simulink model "Testbench_slx_Updated_Presentation"  (R2021a)
settings: Solver=FixedStepAuto  StartTime=0.0  StopTime=0.3  FixedStep=1e-5  RelTol=1e-3
undefined symbols (not defined in the file): D1, Delta
libraries: spsIGBTDiodeLib x52, spsDiodeLib x28, spsSeriesRLCBranchLib x27, spsVariableInductorLib x18, spsGroundLib x7, spsThreePhaseTransformerTwoWindingsLib x6, spsThreePhaseVIMeasurementLib x6, spsAlphaBetaZerotodq0Lib x4, spsVariableCapacitorLib x3, spsVariableResistorLib x3, spsDCVoltageSourceLib x2, pid_lib x2
settings Model: Creator=sjpra  LastModifiedBy=tanmoyera
settings SolverCC: AlgebraicLoopSolver=TrustRegion
settings DebuggingCC: SFMachineParentedDataDiag=warning

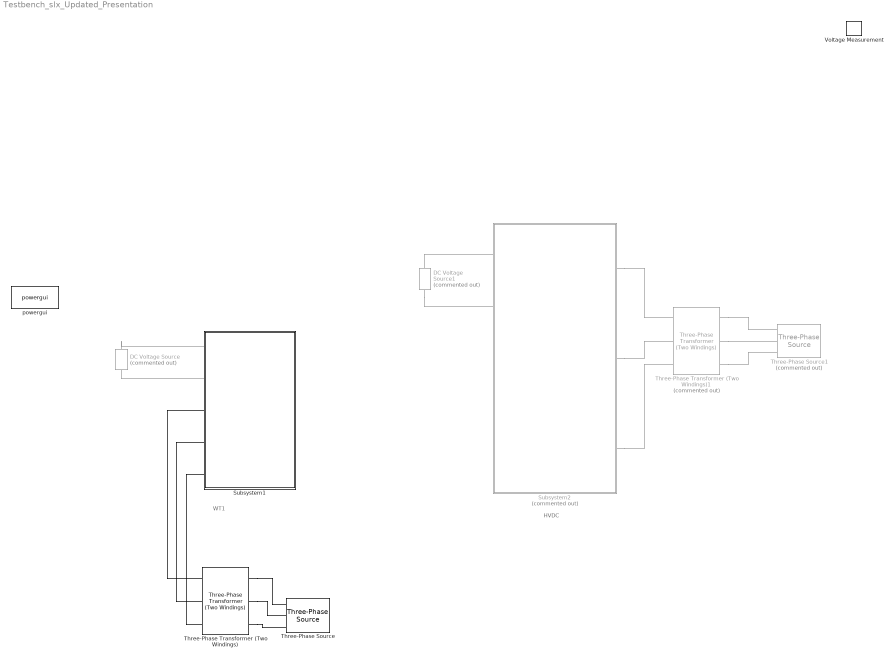
== system Testbench_slx_Updated_Presentation ==
  note: HVDC
  note: WT1
  DC Voltage Source : spsDCVoltageSourceLib/DC Voltage Source  Commented=on  Amplitude=40  Measurements=None
  DC Voltage Source1 : spsDCVoltageSourceLib/DC Voltage Source  Commented=on  Amplitude=40  Measurements=None
  Subsystem1 : Subsystem
  Subsystem2 : Subsystem  Commented=on
  Three-Phase Transformer (Two Windings) : spsThreePhaseTransformerTwoWindingsLib/Three-Phase Transformer (Two Windings)  Winding1Connection=Yg  Winding2Connection=Yg  CoreType=Three single-phase transformers  SetSaturation=off  Hysteresis=off  DataFile='hysteresis'  SetInitialFlux=off  Measurements=None  UNITS=pu  NominalPower=[ 1e3 , 50 ]  Winding1=[ 25 , 0.002 , 0.08 ]  Winding2=[ 400 , 0.002 , 0.08 ]  Rm=500  Lm=500  L0=0.5  Saturation=[ 0,0 ; 0.0024,1.2 ; 1.0,1.52 ]  InitialFluxes=[ 0.8 , -0.8 , 0.7 ]  BreakLoop=off  DiscreteSolver=Trapezoidal iterative  DataType=off  TransfoNumber=1
  Three-Phase Transformer (Two Windings)1 : spsThreePhaseTransformerTwoWindingsLib/Three-Phase Transformer (Two Windings)  Commented=on  Winding1Connection=Yg  Winding2Connection=Yg  CoreType=Three single-phase transformers  SetSaturation=off  Hysteresis=off  DataFile='hysteresis'  SetInitialFlux=off  Measurements=None  UNITS=pu  NominalPower=[ 250e6 , 50 ]  Winding1=[ 25 , 0.002 , 0.08 ]  Winding2=[ 400 , 0.002 , 0.08 ]  Rm=500  Lm=500  L0=0.5  Saturation=[ 0,0 ; 0.0024,1.2 ; 1.0,1.52 ]  InitialFluxes=[ 0.8 , -0.8 , 0.7 ]  BreakLoop=off  DiscreteSolver=Trapezoidal iterative  DataType=off  TransfoNumber=1
  Three-Phase Source : spsThreePhaseSourceLib/Three-Phase Source  InternalConnection=Yg  VoltagePhases=off  Voltage=25e3  PhaseAngle=0  Voltage_phases=[25e3 25e3 25e3]/sqrt(3)  PhaseAngles_phases=[0 -120 +120]  Frequency=50  NonIdealSource=on  SpecifyImpedance=off  Resistance=0.8929  Inductance=16.58e-3  ShortCircuitLevel=100e6  BaseVoltage=25e3  XRratio=7  BusType=swing  Pref=10e3  Qref=0  Prefabc=[10e3, 10e3, 10e3]  Qrefabc=[0, 0, 0]  Qmin=-inf  Qmax=inf
  Three-Phase Source1 : spsThreePhaseSourceLib/Three-Phase Source  Commented=on  InternalConnection=Yg  VoltagePhases=off  Voltage=25e3  PhaseAngle=0  Voltage_phases=[25e3 25e3 25e3]/sqrt(3)  PhaseAngles_phases=[0 -120 +120]  Frequency=50  NonIdealSource=on  SpecifyImpedance=off  Resistance=0.8929  Inductance=16.58e-3  ShortCircuitLevel=100e6  BaseVoltage=25e3  XRratio=7  BusType=swing  Pref=10e3  Qref=0  Prefabc=[10e3, 10e3, 10e3]  Qrefabc=[0, 0, 0]  Qmin=-inf  Qmax=inf
  Voltage Measurement : spsVoltageMeasurementLib/Voltage Measurement  PhasorSimulation=off  OutputType=Complex  PSBequivalent=0
  powergui : spspowerguiLib/powergui  Priority=1  SimulationMode=Discrete  SampleTime=1e-6  frequency=60  Iterations=50  frequencyindice=0  Pbase=1e3  ErrMax=1e-4  UnitsV=V  UnitsW=W  buscounter=0  FunctionMessages=off  echomessages=off  EnableUseOfTLC=off  CurrentSourceSwitches=off  DisableSnubberDevices=off  DisableRonSwitches=off  DisableVfSwitches=off  DisplayEquations=off  AutomaticDiscreteSolvers=off  SolverType=Tustin/Backward Euler (TBE)  Interpol=off  ExternalGateDelay=off  methode=off  Ts=100  x0status=blocks  SPID=on  SwTol=0  HookPort=off  NonlinearTolerance=1e-4  nMaxIteration=100  ContinueOnMaxIteration=off  RestoreLinks=warning  ResistiveCurrentMeasurement=off  Frange=[0:2:500]  Ylog=off  Xlog=on  ShowGrid=off  save=off  variable=ZData  structure=0  ZoomFFT=off  StartTime=0.0  cycles=1  DisplayStyle=1  fundamental=60  FreqAxis=off  MaxFrequency=1000  frequencyindicesteady=1  RmsSteady=1  display=off
  connections:
  DC Voltage Source/RConn1 -- Subsystem1/LConn1
  DC Voltage Source/LConn1 -- Subsystem1/LConn2
  DC Voltage Source1/RConn1 -- Subsystem2/LConn1
  DC Voltage Source1/LConn1 -- Subsystem2/LConn2
  Subsystem1/LConn3 -- Three-Phase Transformer (Two Windings)/LConn1
  Subsystem1/LConn4 -- Three-Phase Transformer (Two Windings)/LConn2
  Subsystem1/LConn5 -- Three-Phase Transformer (Two Windings)/LConn3
  Three-Phase Transformer (Two Windings)/RConn1 -- Three-Phase Source/RConn1
  Three-Phase Transformer (Two Windings)/RConn2 -- Three-Phase Source/RConn2
  Three-Phase Transformer (Two Windings)/RConn3 -- Three-Phase Source/RConn3
  Subsystem2/RConn1 -- Three-Phase Transformer (Two Windings)1/LConn1
  Subsystem2/RConn2 -- Three-Phase Transformer (Two Windings)1/LConn2
  Subsystem2/RConn3 -- Three-Phase Transformer (Two Windings)1/LConn3
  Three-Phase Transformer (Two Windings)1/RConn1 -- Three-Phase Source1/RConn1
  Three-Phase Transformer (Two Windings)1/RConn2 -- Three-Phase Source1/RConn2
  Three-Phase Transformer (Two Windings)1/RConn3 -- Three-Phase Source1/RConn3

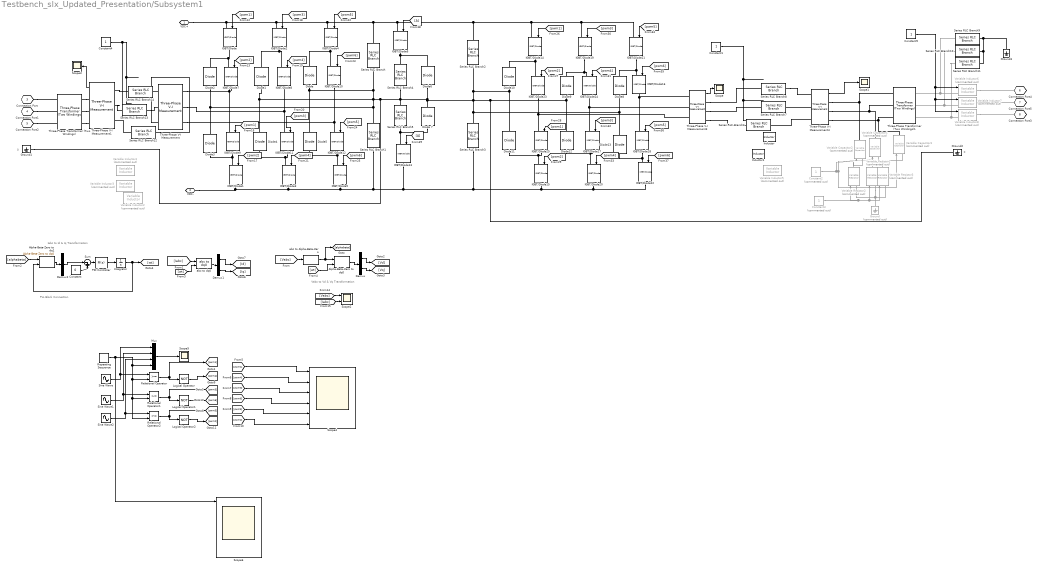
== system Testbench_slx_Updated_Presentation/Subsystem1 ==
  note: 0
  note: 0
  note: Iabc to Id & Iq Transformation
  note: Vabc to Vd & Vq Transformation
  note: PLL Block Connection
  Alpha-Beta-Zero to dq0 : spsAlphaBetaZerotodq0Lib/Alpha-Beta-Zero to dq0  Alignment=90 degrees behind phase A axis
      settings: SourceProductBaseCode=PS
  Alpha-Beta-Zero to dq1 : spsAlphaBetaZerotodq0Lib/Alpha-Beta-Zero to dq0  Alignment=90 degrees behind phase A axis
      settings: SourceProductBaseCode=PS
  Constant : Constant  Value=0
  Constant1 : Constant
  Constant2 : Constant  Commented=on
  Constant3 : Constant  Commented=on
  Constant4 : Constant
  Constant5 : Constant
  Demux : Demux  Outputs=2
  Demux1 : Demux  Outputs=2
  Demux2 : Demux  Outputs=1
  Diode{,1..6,8..13} (13 alike) : spsDiodeLib/Diode  Ron=0.001  Lon=0  Vf=0.8  IC=0  UseSnubber=0  Rs=500  Cs=250e-9  Measurements=off
  Diode 7 : spsDiodeLib/Diode  Ron=0.001  Lon=0  Vf=0.8  IC=0  UseSnubber=0  Rs=500  Cs=250e-9  Measurements=off
  Ground : spsGroundLib/Ground  Commented=on  LConnTagsString=a
  Ground1 : spsGroundLib/Ground  LConnTagsString=a
  Ground2 : spsGroundLib/Ground  LConnTagsString=a
  Ground3 : spsGroundLib/Ground  LConnTagsString=a
  IGBT/Diode{,1..25} (26 alike) : spsIGBTDiodeLib/IGBT//Diode  Ron=1e-3  Rs=1e5  Cs=inf  Measurements=off
  Inductor : fl_lib/Electrical/Electrical Elements/Inductor  l=1e-6 H  r=0 Ohm  g=1e-9 1/Ohm  i_specify=off  i_priority=None  i=0 A  i_nominal_specify=off  i_nominal_unit=A  i_nominal_value=1  v_specify=off  v_priority=None  v=0 V  v_nominal_specify=off  v_nominal_unit=V  v_nominal_value=1  i_L_specify=off  i_L_priority=High  i_L=0 A  i_L_nominal_specify=off  i_L_nominal_unit=A  i_L_nominal_value=1
  Inductor1 : ee_lib/Passive/Inductor  l=1e-6 H  L_tol=20  enable_L_tol=0  tol_distribution=1  nSigma=4  r=0 Ohm  g=1e-9 1/Ohm  enable_operating_limits=0  operating_limit_action=2  max_working_current=1 A  power_rating=1 W  enable_faults=0  fault_action=1  lambdaPercent=50  k_faulted=0.9999  turnsShort=0  openCct=0  groundShort=0  groundShortG=0 1/Ohm  tau_fault=1e-3 s  enable_temporal_fault=0  t_fault=1 s  enable_behavioral_fault=0  max_permissible_voltage=100 V  n_fail_on_voltage=1  max_permissible_current=1 A  t_fail_on_current=1 s  i_L_specify=off  i_L_priority=High  i_L=0 A  i_L_nominal_specify=off  i_L_nominal_unit=A  i_L_nominal_value=1
  Integrator : Integrator
  Logical Operator : Logic  Operator=NOT  AllPortsSameDT=off  OutDataTypeStr=boolean
  Logical Operator1 : Logic  Operator=NOT  AllPortsSameDT=off  OutDataTypeStr=boolean
  Logical Operator2 : Logic  Operator=NOT  AllPortsSameDT=off  OutDataTypeStr=boolean
  Mux : Mux
  PID Controller : pid_lib/PID Controller  Controller=PI  Form=Parallel  TimeDomain=Continuous-time  UseExternalTs=off  SampleTime=-1  IntegratorMethod=Forward Euler  FilterMethod=Forward Euler  ControllerParametersSource=internal  P=10  I=50000  D=0  UseFilter=on  N=100  TunerSelectOption=Transfer Function Based (PID Tuner App)  InitialConditionSource=internal  InitialConditionForIntegrator=0  InitialConditionForFilter=0  DifferentiatorICPrevScaledInput=0  ExternalReset=none  TrackingMode=off  Kt=1  LimitOutput=off  SatLimitsSource=internal  UpperSaturationLimit=inf  LowerSaturationLimit=-inf  LinearizeAsGain=on  AntiWindupMode=none  Kb=1  POutMin=[]  POutMax=[]  IOutMin=[]  IOutMax=[]  DOutMin=[]  DOutMax=[]  NOutMin=[]  NOutMax=[]  SumOutMin=[]  SumOutMax=[]  SaturationOutMin=[]  SaturationOutMax=[]  PParamMin=[]  PParamMax=[]  IParamMin=[]  IParamMax=[]  DParamMin=[]  DParamMax=[]  NParamMin=[]  NParamMax=[]  KbParamMin=[]  KbParamMax=[]  KtParamMin=[]  KtParamMax=[]  KbOutMin=[]  KbOutMax=[]  KtOutMin=[]  KtOutMax=[]  IntegratorOutMin=[]  IntegratorOutMax=[]  FilterOutMin=[]  FilterOutMax=[]  SumI1OutMin=[]  SumI1OutMax=[]  SumI2OutMin=[]  SumI2OutMax=[]  SumI3OutMin=[]  SumI3OutMax=[]  SumI4OutMin=[]  SumI4OutMax=[]  SumDOutMin=[]  SumDOutMax=[]  DifferentiatorOutMin=[]  DifferentiatorOutMax=[]  FilterDiffOutCoefMin=[]  FilterDiffOutCoefMax=[]  ReciprocalOutMin=[]  ReciprocalOutMax=[]  SumDenOutMin=[]  SumDenOutMax=[]  SumNumOutMin=[]  SumNumOutMax=[]  DivideOutMin=[]  DivideOutMax=[]  UdiffTsProdOutMin=[]  UdiffTsProdOutMax=[]  NTsProdOutMin=[]  NTsProdOutMax=[]  UintegralTsProdOutMin=[]  UintegralTsProdOutMax=[]  UngainTsProdOutMin=[]  UngainTsProdOutMax=[]  IntegratorContinuousStateAttributes=''  IntegratorStateMustResolveToSignalObject=off  IntegratorRTWStateStorageClass=Auto  FilterContinuousStateAttributes=''  FilterStateMustResolveToSignalObject=off  FilterRTWStateStorageClass=Auto  ParallelPVariant=InternalParameters  IdealPVariant=Disabled  IVariant=InternalParameters  DVariant=Disabled  IntegratorVariant=Continuous  SatVariant=Disabled  AWVariant=Passthrough  PCopyVariant=Disabled  TRVariant=Disabled  FdbkBlocksVariant=Forward  IdealPFdbkVariant=Disabled  SatFdbkVariant=Disabled  DerivativeFilterVariant=Disabled  NVariant=Disabled  NCopyVariant=Disabled_SignalSpec  FilterICVariant=Disabled  IntegratorICVariant=InternalICs  ExternalResetVariant=Disabled  TRSumVariant=Passthrough  SumFdbkVariant=Disabled  SumVariant=Sum_PI  TsampFilterVariant=InternalTs  TsampNgainVariant=Passthrough  TsampIntegralVariant=Passthrough  ExternalSaturationOutDataTypeStr=Inherit: Same as second input
  Relational Operator : RelationalOperator  OutDataTypeStr=boolean  RndMeth=Simplest
  Relational Operator1 : RelationalOperator  OutDataTypeStr=boolean  RndMeth=Simplest
  Relational Operator2 : RelationalOperator  OutDataTypeStr=boolean  RndMeth=Simplest
  Repeating Sequence : simulink/Sources/Repeating Sequence  rep_seq_t=[0 1 2 3]*[1/6000]  rep_seq_y=[0 1 -1 0]
  Scope{,1,3,5} (4 alike) : Scope
  Scope2 : Scope  NumInputPorts=2
  Scope4 : Scope  NumInputPorts=6
  Scope6 : Scope  NumInputPorts=6
  Series RLC Branch{,1..3} (4 alike) : spsSeriesRLCBranchLib/Series RLC Branch  LConnTagsString=__new0  RConnTagsString=__new0  BranchType=C  Resistance=1  Inductance=1e-3  SetiL0=off  InitialCurrent=0  Capacitance=26e-6  Setx0=off  InitialVoltage=0  Measurements=None
  Series RLC Branch10 : spsSeriesRLCBranchLib/Series RLC Branch  LConnTagsString=__new0  RConnTagsString=__new0  BranchType=R  Resistance=1e6  Inductance=1e-3  SetiL0=off  InitialCurrent=0  Capacitance=1e-6  Setx0=off  InitialVoltage=0  Measurements=None
  Series RLC Branch11 : spsSeriesRLCBranchLib/Series RLC Branch  LConnTagsString=__new0  RConnTagsString=__new0  BranchType=R  Resistance=1e6  Inductance=1e-3  SetiL0=off  InitialCurrent=0  Capacitance=1e-6  Setx0=off  InitialVoltage=0  Measurements=None
  Series RLC Branch{6..8,12..14} (6 alike) : spsSeriesRLCBranchLib/Series RLC Branch  LConnTagsString=__new0  RConnTagsString=__new0  BranchType=L  Resistance=1  Inductance=1e-3  SetiL0=off  InitialCurrent=0  Capacitance=1e-6  Setx0=off  InitialVoltage=0  Measurements=None
  Series RLC Branch4 : spsSeriesRLCBranchLib/Series RLC Branch  LConnTagsString=__new0  RConnTagsString=__new0  BranchType=R  Resistance=1  Inductance=1e-3  SetiL0=off  InitialCurrent=0  Capacitance=1e-6  Setx0=off  InitialVoltage=0  Measurements=None
  Series RLC Branch5 : spsSeriesRLCBranchLib/Series RLC Branch  LConnTagsString=__new0  RConnTagsString=__new0  BranchType=R  Resistance=1  Inductance=1e-3  SetiL0=off  InitialCurrent=0  Capacitance=1e-6  Setx0=off  InitialVoltage=0  Measurements=None
  Series RLC Branch9 : spsSeriesRLCBranchLib/Series RLC Branch  LConnTagsString=__new0  RConnTagsString=__new0  BranchType=R  Resistance=1e6  Inductance=1e-3  SetiL0=off  InitialCurrent=0  Capacitance=1e-6  Setx0=off  InitialVoltage=0  Measurements=None
  Sine Wave : Sin  Frequency=2*pi*50  SampleTime=0
  Sine Wave1 : Sin  Frequency=2*pi*50  Phase=2*pi/3  SampleTime=0
  Sine Wave2 : Sin  Frequency=2*pi*50  Phase=-2*pi/3  SampleTime=0
  Sum : Sum  Inputs=|-+
  Three-Phase Transformer (Two Windings) : spsThreePhaseTransformerTwoWindingsLib/Three-Phase Transformer (Two Windings)  Winding1Connection=Delta (D1)  Winding2Connection=Yg  CoreType=Three single-phase transformers  SetSaturation=off  Hysteresis=off  DataFile='hysteresis'  SetInitialFlux=off  Measurements=None  UNITS=pu  NominalPower=[ 1e3 , 50 ]  Winding1=[ 735e3 , 0.002 , 0.08 ]  Winding2=[ 315e3 , 0.002 , 0.08 ]  Rm=500  Lm=500  L0=0.5  Saturation=[ 0,0 ; 0.0024,1.2 ; 1.0,1.52 ]  InitialFluxes=[ 0.8 , -0.8 , 0.7 ]  BreakLoop=off  DiscreteSolver=Trapezoidal iterative  DataType=off  TransfoNumber=1
  Three-Phase Transformer (Two Windings)1 : spsThreePhaseTransformerTwoWindingsLib/Three-Phase Transformer (Two Windings)  Winding1Connection=Yg  Winding2Connection=Delta (D1)  CoreType=Three single-phase transformers  SetSaturation=off  Hysteresis=off  DataFile='hysteresis'  SetInitialFlux=off  Measurements=None  UNITS=pu  NominalPower=[ 1e3 , 50 ]  Winding1=[ 735e3 , 0.002 , 0.08 ]  Winding2=[ 315e3 , 0.002 , 0.08 ]  Rm=500  Lm=500  L0=0.5  Saturation=[ 0,0 ; 0.0024,1.2 ; 1.0,1.52 ]  InitialFluxes=[ 0.8 , -0.8 , 0.7 ]  BreakLoop=off  DiscreteSolver=Trapezoidal iterative  DataType=off  TransfoNumber=1
  Three-Phase V-I Measurement : spsThreePhaseVIMeasurementLib/Three-Phase V-I Measurement  VoltageMeasurement=no  SetLabelV=off  LabelV=Vabc  Vpu=off  VpuLL=off  CurrentMeasurement=yes  SetLabelI=on  LabelI=IRYB  Ipu=on  Pbase=1e3  Vbase=25  OutputType=Complex  PhasorSimulation=off  PSBequivalent=0
  Three-Phase V-I Measurement1 : spsThreePhaseVIMeasurementLib/Three-Phase V-I Measurement  VoltageMeasurement=phase-to-phase  SetLabelV=off  LabelV=Vabc  Vpu=off  VpuLL=on  CurrentMeasurement=no  SetLabelI=off  LabelI=IRYB  Ipu=off  Pbase=100e6  Vbase=25  OutputType=Complex  PhasorSimulation=off  PSBequivalent=0
  Three-Phase V-I Measurement3 : spsThreePhaseVIMeasurementLib/Three-Phase V-I Measurement  VoltageMeasurement=no  SetLabelV=off  LabelV=Vabc  Vpu=off  VpuLL=off  CurrentMeasurement=yes  SetLabelI=off  LabelI=IRYB  Ipu=off  Pbase=100e6  Vbase=500e3  OutputType=Complex  PhasorSimulation=off  PSBequivalent=0
  Three-Phase V-I Measurement4 : spsThreePhaseVIMeasurementLib/Three-Phase V-I Measurement  VoltageMeasurement=phase-to-phase  SetLabelV=off  LabelV=Vabc  Vpu=off  VpuLL=off  CurrentMeasurement=no  SetLabelI=off  LabelI=IRYB  Ipu=off  Pbase=100e6  Vbase=500e3  OutputType=Complex  PhasorSimulation=off  PSBequivalent=0
  Variable Capacitor1 : spsVariableCapacitorLib/Variable Capacitor  Commented=on  methode=Backward Euler  Cabsmin=235e-6  Initialize=off  vC0=0  C0=1e-6  iC0=0
      settings: SourceProductBaseCode=PS
  Variable Capacitor2 : spsVariableCapacitorLib/Variable Capacitor  Commented=on  methode=Backward Euler  Cabsmin=235e-6  Initialize=off  vC0=0  C0=1e-6  iC0=0
      settings: SourceProductBaseCode=PS
  Variable Capacitor3 : spsVariableCapacitorLib/Variable Capacitor  Commented=on  methode=Backward Euler  Cabsmin=235e-6  Initialize=off  vC0=0  C0=1e-6  iC0=0
      settings: SourceProductBaseCode=PS
  Variable Inductor{2..8} (7 alike) : spsVariableInductorLib/Variable Inductor  Commented=on  methode=Trapezoidal  Labsmin=0.1e-3  Initialize=off  iL0=0  L0=1e-3  Vl0=0
      settings: SourceProductBaseCode=PS
  Variable Resistor1 : spsVariableResistorLib/Variable Resistor  Commented=on  Rabsmin=0.3
      settings: SourceProductBaseCode=PS
  Variable Resistor2 : spsVariableResistorLib/Variable Resistor  Commented=on  Rabsmin=0.3
      settings: SourceProductBaseCode=PS
  Variable Resistor3 : spsVariableResistorLib/Variable Resistor  Commented=on  Rabsmin=0.3
      settings: SourceProductBaseCode=PS
  abc to Alpha-Beta-Zero : spsabctoAlphaBetaZeroLib/abc to Alpha-Beta-Zero
      settings: SourceProductBaseCode=PS
  abc to dq0 : spsabctodq0Lib/abc to dq0  Alignment=90 degrees behind phase A axis
  VDC+ : PMIOPort  Side=Left
  VDC- : PMIOPort  Port=2  Side=Left
  Connection Port : PMIOPort  Tag=PMCPort  Port=3  Side=Left
  Connection Port1 : PMIOPort  Tag=PMCPort  Port=4  Side=Left
  Connection Port2 : PMIOPort  Tag=PMCPort  Port=5  Side=Left
  Connection Port4 : PMIOPort  Tag=PMCPort  Port=6  Side=Right
  Connection Port5 : PMIOPort  Tag=PMCPort  Port=7  Side=Right
  Connection Port3 : PMIOPort  Tag=PMCPort  Port=8  Side=Right
  wires:
  [pwm6] -> IGBT/Diode5/1
  [pwm6] -> IGBT/Diode10/1
  [pwm1] -> IGBT/Diode/1
  [pwm2] -> IGBT/Diode1/1
  [pwm1] -> IGBT/Diode9/1
  [pwm4] -> IGBT/Diode3/1
  [pwm2] -> IGBT/Diode7/1
  [pwm3] -> IGBT/Diode2/1
  [pwm5] -> IGBT/Diode4/1
  [pwm4] -> IGBT/Diode8/1
  [pwm3] -> IGBT/Diode11/1
  [pwm5] -> IGBT/Diode12/1
  [pwm5] -> IGBT/Diode18/1
  [pwm3] -> IGBT/Diode17/1
  [pwm4] -> IGBT/Diode24/1
  [pwm5] -> IGBT/Diode21/1
  [pwm3] -> IGBT/Diode19/1
  [pwm2] -> IGBT/Diode23/1
  [pwm4] -> IGBT/Diode20/1
  [pwm1] -> IGBT/Diode25/1
  [pwm2] -> IGBT/Diode15/1
  [pwm1] -> IGBT/Diode14/1
  [pwm6] -> IGBT/Diode16/1
  [pwm6] -> IGBT/Diode22/1
  Three-Phase V-I Measurement3/1 -> Scope/1
  Three-Phase V-I Measurement4/1 -> Scope1/1
  abc to Alpha-Beta-Zero/1 -> Alpha-Beta-Zero to dq0/1, [alphabeta]
  [Vabc] -> abc to Alpha-Beta-Zero/1
  Alpha-Beta-Zero to dq0/1 -> Demux/1
  Demux/2 -> [Vq]
  [Iabc] -> abc to dq0/1
  abc to dq0/1 -> Demux1/1
  Demux1/2 -> [Iq]
  [alphabeta] -> Alpha-Beta-Zero to dq1/1
  Alpha-Beta-Zero to dq1/1 -> Demux2/1
  Demux2/1 -> Sum/1
  Constant/1 -> Sum/2
  Sum/1 -> PID Controller/1
  PID Controller/1 -> Integrator/1
  Integrator/1 -> [wt], Alpha-Beta-Zero to dq1/2
  [wt] -> abc to dq0/2
  [wt] -> Alpha-Beta-Zero to dq0/2
  [Vabc] -> Scope2/1
  [Iabc] -> Scope2/2
  Three-Phase V-I Measurement1/1 -> Scope3/1
  Demux/1 -> [Vd]
  Demux1/1 -> [Id]
  [A] -> IGBT/Diode6/1
  [A] -> IGBT/Diode13/1
  [pwm6] -> Scope4/4
  [pwm4] -> Scope4/2
  Repeating Sequence/1 -> Scope6/1, Relational Operator/2, Relational Operator1/2, Relational Operator2/2, Mux/4
  Sine Wave2/1 -> Mux/3, Relational Operator2/1
  Relational Operator/1 -> Logical Operator/1, [pwm1]
  Logical Operator2/1 -> [pwm2]
  Mux/1 -> Scope5/1
  Logical Operator1/1 -> [pwm6]
  Sine Wave/1 -> Relational Operator/1, Mux/1
  Relational Operator2/1 -> [pwm5], Logical Operator2/1
  Sine Wave1/1 -> Relational Operator1/1, Mux/2
  [pwm5] -> Scope4/5
  [pwm2] -> Scope4/6
  [pwm3] -> Scope4/3
  [pwm1] -> Scope4/1
  Logical Operator/1 -> [pwm4]
  Relational Operator1/1 -> [pwm3], Logical Operator1/1
  Constant1/1 -> ?
  Constant2/1 -> Variable Capacitor3/1, Variable Capacitor1/1, Variable Capacitor2/1
  Constant3/1 -> Variable Resistor3/1, Variable Resistor1/1, Variable Resistor2/1
  Constant4/1 -> ?
  Constant5/1 -> Variable Inductor8/1, Variable Inductor7/1, Variable Inductor6/1
  connections:
  IGBT/Diode9/RConn1 -- Diode3/LConn1 -- IGBT/Diode1/LConn1
  IGBT/Diode2/RConn1 -- Diode1/RConn1 -- IGBT/Diode8/LConn1
  IGBT/Diode7/RConn1 -- IGBT/Diode9/LConn1 -- Three-Phase V-I Measurement/RConn1
  IGBT/Diode1/RConn1 -- VDC-/RConn1 -- IGBT/Diode3/RConn1 -- Series RLC Branch1/RConn1 -- IGBT/Diode13/RConn1 -- Series RLC Branch3/RConn1 -- IGBT/Diode22/RConn1 -- IGBT/Diode20/RConn1 -- IGBT/Diode15/RConn1 -- IGBT/Diode5/RConn1
  IGBT/Diode10/RConn1 -- IGBT/Diode12/LConn1 -- Three-Phase V-I Measurement/RConn3
  IGBT/Diode11/RConn1 -- Diode4/LConn1 -- IGBT/Diode3/LConn1
  IGBT/Diode12/RConn1 -- Diode5/LConn1 -- IGBT/Diode5/LConn1
  IGBT/Diode7/LConn1 -- IGBT/Diode/RConn1 -- Diode2/RConn1
  IGBT/Diode4/RConn1 -- Diode/RConn1 -- IGBT/Diode10/LConn1
  IGBT/Diode11/LConn1 -- IGBT/Diode8/RConn1 -- Three-Phase V-I Measurement/RConn2
  IGBT/Diode6/RConn1 -- Diode6/RConn1 -- Series RLC Branch4/LConn1
  IGBT/Diode13/LConn1 -- Diode 7/LConn1 -- Series RLC Branch5/RConn1
  Diode11/LConn1 -- IGBT/Diode15/LConn1 -- IGBT/Diode25/RConn1
  Diode9/RConn1 -- IGBT/Diode19/RConn1 -- IGBT/Diode24/LConn1
  IGBT/Diode23/RConn1 -- IGBT/Diode25/LConn1 -- Three-Phase V-I Measurement3/LConn3
  IGBT/Diode18/LConn1 -- IGBT/Diode16/RConn1 -- Three-Phase V-I Measurement3/LConn1
  Diode12/LConn1 -- IGBT/Diode20/LConn1 -- IGBT/Diode17/RConn1
  IGBT/Diode/LConn1 -- VDC+/RConn1 -- Series RLC Branch2/LConn1 -- IGBT/Diode14/LConn1 -- IGBT/Diode21/LConn1 -- IGBT/Diode19/LConn1 -- IGBT/Diode6/LConn1 -- Series RLC Branch/LConn1 -- IGBT/Diode4/LConn1 -- IGBT/Diode2/LConn1
  Diode13/LConn1 -- IGBT/Diode18/RConn1 -- IGBT/Diode22/LConn1
  IGBT/Diode14/RConn1 -- IGBT/Diode23/LConn1 -- Diode10/RConn1
  Diode8/RConn1 -- IGBT/Diode21/RConn1 -- IGBT/Diode16/LConn1
  IGBT/Diode17/LConn1 -- Three-Phase V-I Measurement3/LConn2 -- IGBT/Diode24/RConn1
  Three-Phase V-I Measurement/LConn1 -- Series RLC Branch14/RConn1
  Series RLC Branch13/RConn1 -- Three-Phase V-I Measurement/LConn2
  Series RLC Branch12/RConn1 -- Three-Phase V-I Measurement/LConn3
  Three-Phase V-I Measurement1/LConn1 -- Series RLC Branch14/LConn1
  Three-Phase V-I Measurement1/LConn2 -- Series RLC Branch13/LConn1
  Series RLC Branch12/LConn1 -- Three-Phase V-I Measurement1/LConn3
  Three-Phase Transformer (Two Windings)/RConn1 -- Three-Phase V-I Measurement1/RConn1
  Three-Phase Transformer (Two Windings)/RConn2 -- Three-Phase V-I Measurement1/RConn2
  Three-Phase Transformer (Two Windings)/RConn3 -- Three-Phase V-I Measurement1/RConn3
  Three-Phase V-I Measurement4/LConn2 -- Series RLC Branch7/RConn1
  Three-Phase V-I Measurement4/LConn3 -- Series RLC Branch6/RConn1
  Series RLC Branch8/RConn1 -- Three-Phase V-I Measurement4/LConn1
  Three-Phase V-I Measurement4/RConn1 -- Three-Phase Transformer (Two Windings)1/LConn1 -- Variable Capacitor2/RConn1
  Three-Phase V-I Measurement4/RConn2 -- Three-Phase Transformer (Two Windings)1/LConn2 -- Variable Capacitor1/RConn1
  Three-Phase V-I Measurement4/RConn3 -- Variable Capacitor3/RConn1 -- Three-Phase Transformer (Two Windings)1/LConn3
  Connection Port/RConn1 -- Three-Phase Transformer (Two Windings)/LConn1
  Connection Port1/RConn1 -- Three-Phase Transformer (Two Windings)/LConn2
  Connection Port2/RConn1 -- Three-Phase Transformer (Two Windings)/LConn3
  Variable Resistor1/RConn1 -- Variable Capacitor1/LConn1
  Variable Resistor3/RConn1 -- Variable Capacitor3/LConn1
  Variable Resistor2/RConn1 -- Variable Capacitor2/LConn1
  Variable Resistor2/LConn1 -- Variable Resistor3/LConn1 -- Ground/LConn1 -- Variable Resistor1/LConn1
  Diode13/RConn1 -- Diode8/LConn1 -- Diode12/RConn1 -- Diode9/LConn1 -- Ground2/LConn1 -- Series RLC Branch5/LConn1 -- Series RLC Branch4/RConn1 -- Ground1/LConn1 -- Diode3/RConn1 -- Diode2/LConn1 -- Series RLC Branch1/LConn1 -- Diode5/RConn1 -- Diode/LConn1 -- Series RLC Branch/RConn1 -- Diode1/LConn1 -- Diode4/RConn1 -- Diode6/LConn1 -- Diode 7/RConn1 -- Series RLC Branch2/RConn1 -- Diode11/RConn1 -- Diode10/LConn1 -- Series RLC Branch3/LConn1
  Three-Phase V-I Measurement3/RConn1 -- Series RLC Branch8/LConn1
  Three-Phase V-I Measurement3/RConn2 -- Series RLC Branch7/LConn1
  Three-Phase V-I Measurement3/RConn3 -- Series RLC Branch6/LConn1
  Variable Inductor6/LConn1 -- Series RLC Branch9/LConn1 -- Three-Phase Transformer (Two Windings)1/RConn1
  Variable Inductor7/LConn1 -- Series RLC Branch10/LConn1 -- Three-Phase Transformer (Two Windings)1/RConn2
  Variable Inductor8/LConn1 -- Series RLC Branch11/LConn1 -- Three-Phase Transformer (Two Windings)1/RConn3
  Variable Inductor6/RConn1 -- Connection Port4/RConn1
  Variable Inductor7/RConn1 -- Connection Port5/RConn1
  Variable Inductor8/RConn1 -- Connection Port3/RConn1
  Series RLC Branch9/RConn1 -- Series RLC Branch10/RConn1 -- Series RLC Branch11/RConn1 -- Ground3/LConn1

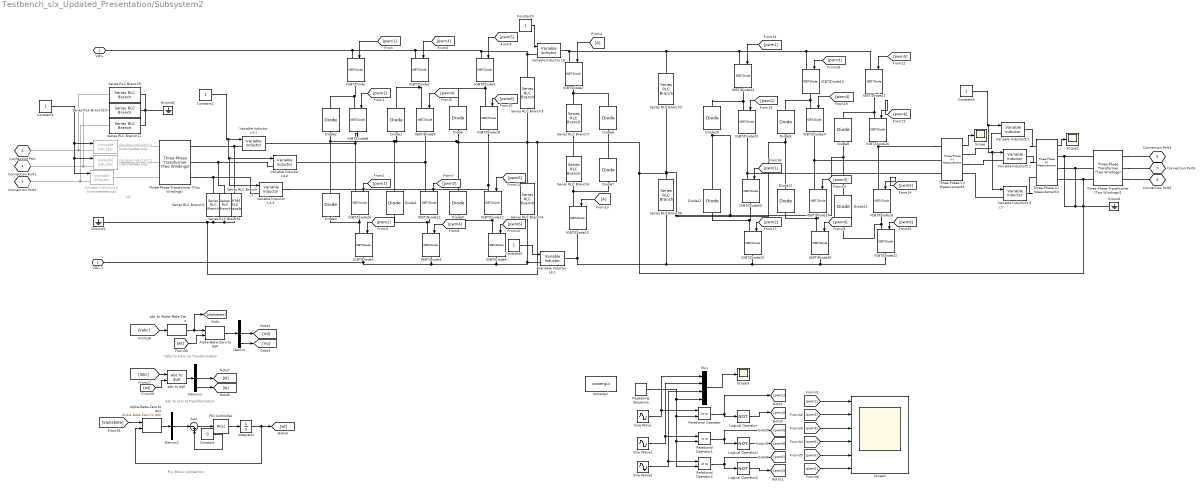
== system Testbench_slx_Updated_Presentation/Subsystem2 ==
  note: L5
  note: L4
  note: L3
  note: Vabc to Vd & Vq Transformation
  note: Iabc to Id & Iq Transformation
  note: PLL Block Connection
  Alpha-Beta-Zero to dq0 : spsAlphaBetaZerotodq0Lib/Alpha-Beta-Zero to dq0  Alignment=90 degrees behind phase A axis
      settings: SourceProductBaseCode=PS
  Alpha-Beta-Zero to dq1 : spsAlphaBetaZerotodq0Lib/Alpha-Beta-Zero to dq0  Alignment=90 degrees behind phase A axis
      settings: SourceProductBaseCode=PS
  Constant : Constant  Value=0
  Constant{1..5} (5 alike) : Constant
  Demux : Demux  Outputs=3
  Demux1 : Demux  Outputs=3
  Demux2 : Demux  Outputs=3
  Diode{,1..13} (14 alike) : spsDiodeLib/Diode  Ron=0.001  Lon=0  Vf=0.8  IC=0  UseSnubber=0  Rs=500  Cs=250e-9  Measurements=off
  Ground : spsGroundLib/Ground  LConnTagsString=a
  Ground1 : spsGroundLib/Ground  LConnTagsString=a
  Ground2 : spsGroundLib/Ground  LConnTagsString=a
  IGBT/Diode{,1..5,7..26} (26 alike) : spsIGBTDiodeLib/IGBT//Diode  Ron=1e-3  Rs=1e5  Cs=inf  Measurements=off
  Integrator : Integrator
  Logical Operator : Logic  Operator=NOT  AllPortsSameDT=off  OutDataTypeStr=boolean
  Logical Operator1 : Logic  Operator=NOT  AllPortsSameDT=off  OutDataTypeStr=boolean
  Logical Operator2 : Logic  Operator=NOT  AllPortsSameDT=off  OutDataTypeStr=boolean
  Mux : Mux
  PID Controller : pid_lib/PID Controller  Controller=PI  Form=Parallel  TimeDomain=Continuous-time  UseExternalTs=off  SampleTime=-1  IntegratorMethod=Forward Euler  FilterMethod=Forward Euler  ControllerParametersSource=internal  P=10  I=50000  D=0  UseFilter=on  N=100  TunerSelectOption=Transfer Function Based (PID Tuner App)  InitialConditionSource=internal  InitialConditionForIntegrator=0  InitialConditionForFilter=0  DifferentiatorICPrevScaledInput=0  ExternalReset=none  TrackingMode=off  Kt=1  LimitOutput=off  SatLimitsSource=internal  UpperSaturationLimit=inf  LowerSaturationLimit=-inf  LinearizeAsGain=on  AntiWindupMode=none  Kb=1  POutMin=[]  POutMax=[]  IOutMin=[]  IOutMax=[]  DOutMin=[]  DOutMax=[]  NOutMin=[]  NOutMax=[]  SumOutMin=[]  SumOutMax=[]  SaturationOutMin=[]  SaturationOutMax=[]  PParamMin=[]  PParamMax=[]  IParamMin=[]  IParamMax=[]  DParamMin=[]  DParamMax=[]  NParamMin=[]  NParamMax=[]  KbParamMin=[]  KbParamMax=[]  KtParamMin=[]  KtParamMax=[]  KbOutMin=[]  KbOutMax=[]  KtOutMin=[]  KtOutMax=[]  IntegratorOutMin=[]  IntegratorOutMax=[]  FilterOutMin=[]  FilterOutMax=[]  SumI1OutMin=[]  SumI1OutMax=[]  SumI2OutMin=[]  SumI2OutMax=[]  SumI3OutMin=[]  SumI3OutMax=[]  SumI4OutMin=[]  SumI4OutMax=[]  SumDOutMin=[]  SumDOutMax=[]  DifferentiatorOutMin=[]  DifferentiatorOutMax=[]  FilterDiffOutCoefMin=[]  FilterDiffOutCoefMax=[]  ReciprocalOutMin=[]  ReciprocalOutMax=[]  SumDenOutMin=[]  SumDenOutMax=[]  SumNumOutMin=[]  SumNumOutMax=[]  DivideOutMin=[]  DivideOutMax=[]  UdiffTsProdOutMin=[]  UdiffTsProdOutMax=[]  NTsProdOutMin=[]  NTsProdOutMax=[]  UintegralTsProdOutMin=[]  UintegralTsProdOutMax=[]  UngainTsProdOutMin=[]  UngainTsProdOutMax=[]  IntegratorContinuousStateAttributes=''  IntegratorStateMustResolveToSignalObject=off  IntegratorRTWStateStorageClass=Auto  FilterContinuousStateAttributes=''  FilterStateMustResolveToSignalObject=off  FilterRTWStateStorageClass=Auto  ParallelPVariant=InternalParameters  IdealPVariant=Disabled  IVariant=InternalParameters  DVariant=Disabled  IntegratorVariant=Continuous  SatVariant=Disabled  AWVariant=Passthrough  PCopyVariant=Disabled  TRVariant=Disabled  FdbkBlocksVariant=Forward  IdealPFdbkVariant=Disabled  SatFdbkVariant=Disabled  DerivativeFilterVariant=Disabled  NVariant=Disabled  NCopyVariant=Disabled_SignalSpec  FilterICVariant=Disabled  IntegratorICVariant=InternalICs  ExternalResetVariant=Disabled  TRSumVariant=Passthrough  SumFdbkVariant=Disabled  SumVariant=Sum_PI  TsampFilterVariant=InternalTs  TsampNgainVariant=Passthrough  TsampIntegralVariant=Passthrough  ExternalSaturationOutDataTypeStr=Inherit: Same as second input
  Relational Operator : RelationalOperator  OutDataTypeStr=boolean  RndMeth=Simplest
  Relational Operator1 : RelationalOperator  OutDataTypeStr=boolean  RndMeth=Simplest
  Relational Operator2 : RelationalOperator  OutDataTypeStr=boolean  RndMeth=Simplest
  Repeating Sequence : simulink/Sources/Repeating Sequence  rep_seq_t=[0 1 2 3]*[1/6000]  rep_seq_y=[0 1 -1 0]
  Scope : Scope
  Scope1 : Scope
  Scope2 : Scope  NumInputPorts=6
  Scope3 : Scope
  Series RLC Branch : spsSeriesRLCBranchLib/Series RLC Branch  LConnTagsString=__new0  RConnTagsString=__new0  BranchType=C  Resistance=1  Inductance=1e-3  SetiL0=off  InitialCurrent=0  Capacitance=1e-6  Setx0=off  InitialVoltage=0  Measurements=None
  Series RLC Branch1 : spsSeriesRLCBranchLib/Series RLC Branch  LConnTagsString=__new0  RConnTagsString=__new0  BranchType=C  Resistance=1  Inductance=1e-3  SetiL0=off  InitialCurrent=0  Capacitance=1e-6  Setx0=off  InitialVoltage=0  Measurements=None
  Series RLC Branch10 : spsSeriesRLCBranchLib/Series RLC Branch  LConnTagsString=__new0  RConnTagsString=__new0  BranchType=R  Resistance=1e6  Inductance=1e-3  SetiL0=off  InitialCurrent=0  Capacitance=1e-6  Setx0=off  InitialVoltage=0  Measurements=None
  Series RLC Branch11 : spsSeriesRLCBranchLib/Series RLC Branch  LConnTagsString=__new0  RConnTagsString=__new0  BranchType=R  Resistance=1e6  Inductance=1e-3  SetiL0=off  InitialCurrent=0  Capacitance=1e-6  Setx0=off  InitialVoltage=0  Measurements=None
  Series RLC Branch2 : spsSeriesRLCBranchLib/Series RLC Branch  LConnTagsString=__new0  RConnTagsString=__new0  BranchType=C  Resistance=1  Inductance=1e-3  SetiL0=off  InitialCurrent=0  Capacitance=1e-6  Setx0=off  InitialVoltage=0  Measurements=None
  Series RLC Branch{3..6} (4 alike) : spsSeriesRLCBranchLib/Series RLC Branch  LConnTagsString=__new0  RConnTagsString=__new0  BranchType=C  Resistance=1  Inductance=1e-3  SetiL0=off  InitialCurrent=0  Capacitance=26e-6  Setx0=off  InitialVoltage=0  Measurements=None
  Series RLC Branch7 : spsSeriesRLCBranchLib/Series RLC Branch  LConnTagsString=__new0  RConnTagsString=__new0  BranchType=R  Resistance=1  Inductance=1e-3  SetiL0=off  InitialCurrent=0  Capacitance=1e-6  Setx0=off  InitialVoltage=0  Measurements=None
  Series RLC Branch8 : spsSeriesRLCBranchLib/Series RLC Branch  LConnTagsString=__new0  RConnTagsString=__new0  BranchType=R  Resistance=1  Inductance=1e-3  SetiL0=off  InitialCurrent=0  Capacitance=1e-6  Setx0=off  InitialVoltage=0  Measurements=None
  Series RLC Branch9 : spsSeriesRLCBranchLib/Series RLC Branch  LConnTagsString=__new0  RConnTagsString=__new0  BranchType=R  Resistance=1e6  Inductance=1e-3  SetiL0=off  InitialCurrent=0  Capacitance=1e-6  Setx0=off  InitialVoltage=0  Measurements=None
  Sine Wave : Sin  Frequency=2*pi*50  SampleTime=0
  Sine Wave1 : Sin  Frequency=2*pi*50  Phase=2*pi/3  SampleTime=0
  Sine Wave2 : Sin  Frequency=2*pi*50  Phase=-2*pi/3  SampleTime=0
  Sum : Sum  Inputs=|-+
  Three-Phase Transformer (Two Windings) : spsThreePhaseTransformerTwoWindingsLib/Three-Phase Transformer (Two Windings)  Winding1Connection=Delta (D1)  Winding2Connection=Y  CoreType=Three single-phase transformers  SetSaturation=off  Hysteresis=off  DataFile='hysteresis'  SetInitialFlux=off  Measurements=None  UNITS=pu  NominalPower=[ 250e6 , 60 ]  Winding1=[ 735e3 , 0.002 , 0.08 ]  Winding2=[ 315e3 , 0.002 , 0.08 ]  Rm=500  Lm=500  L0=0.5  Saturation=[ 0,0 ; 0.0024,1.2 ; 1.0,1.52 ]  InitialFluxes=[ 0.8 , -0.8 , 0.7 ]  BreakLoop=off  DiscreteSolver=Trapezoidal iterative  DataType=off  TransfoNumber=1
  Three-Phase Transformer (Two Windings)1 : spsThreePhaseTransformerTwoWindingsLib/Three-Phase Transformer (Two Windings)  Winding1Connection=Yg  Winding2Connection=Delta (D1)  CoreType=Three single-phase transformers  SetSaturation=off  Hysteresis=off  DataFile='hysteresis'  SetInitialFlux=off  Measurements=None  UNITS=pu  NominalPower=[ 250e6 , 60 ]  Winding1=[ 735e3 , 0.002 , 0.08 ]  Winding2=[ 315e3 , 0.002 , 0.08 ]  Rm=500  Lm=500  L0=0.5  Saturation=[ 0,0 ; 0.0024,1.2 ; 1.0,1.52 ]  InitialFluxes=[ 0.8 , -0.8 , 0.7 ]  BreakLoop=off  DiscreteSolver=Trapezoidal iterative  DataType=off  TransfoNumber=1
  Three-Phase V-I Measurement3 : spsThreePhaseVIMeasurementLib/Three-Phase V-I Measurement  VoltageMeasurement=no  SetLabelV=off  LabelV=Vabc  Vpu=off  VpuLL=off  CurrentMeasurement=yes  SetLabelI=off  LabelI=IRYB  Ipu=off  Pbase=100e6  Vbase=500e3  OutputType=Complex  PhasorSimulation=off  PSBequivalent=0
  Three-Phase V-I Measurement4 : spsThreePhaseVIMeasurementLib/Three-Phase V-I Measurement  VoltageMeasurement=phase-to-phase  SetLabelV=off  LabelV=Vabc  Vpu=off  VpuLL=off  CurrentMeasurement=no  SetLabelI=off  LabelI=IRYB  Ipu=off  Pbase=100e6  Vbase=500e3  OutputType=Complex  PhasorSimulation=off  PSBequivalent=0
  Variable Inductor L4.1 : spsVariableInductorLib/Variable Inductor  methode=Trapezoidal  Labsmin=0.1e-3  Initialize=off  iL0=0  L0=1e-3  Vl0=0
      settings: SourceProductBaseCode=PS
  Variable Inductor L4.2 : spsVariableInductorLib/Variable Inductor  methode=Trapezoidal  Labsmin=0.1e-3  Initialize=off  iL0=0  L0=1e-3  Vl0=0
      settings: SourceProductBaseCode=PS
  Variable Inductor L4.3 : spsVariableInductorLib/Variable Inductor  methode=Trapezoidal  Labsmin=0.1e-3  Initialize=off  iL0=0  L0=1e-3  Vl0=0
      settings: SourceProductBaseCode=PS
  Variable Inductor L6 : spsVariableInductorLib/Variable Inductor  methode=Backward Euler  Labsmin=0.1e-3  Initialize=off  iL0=0  L0=1e-3  Vl0=0
      settings: SourceProductBaseCode=PS
  Variable Inductor L6.1 : spsVariableInductorLib/Variable Inductor  methode=Backward Euler  Labsmin=0.1e-3  Initialize=off  iL0=0  L0=1e-3  Vl0=0
      settings: SourceProductBaseCode=PS
  Variable Inductor5.1 : spsVariableInductorLib/Variable Inductor  methode=Trapezoidal  Labsmin=0.1e-3  Initialize=off  iL0=0  L0=1e-3  Vl0=0
      settings: SourceProductBaseCode=PS
  Variable Inductor5.2 : spsVariableInductorLib/Variable Inductor  methode=Trapezoidal  Labsmin=0.1e-3  Initialize=off  iL0=0  L0=1e-3  Vl0=0
      settings: SourceProductBaseCode=PS
  Variable Inductor5.3 : spsVariableInductorLib/Variable Inductor  methode=Trapezoidal  Labsmin=0.1e-3  Initialize=off  iL0=0  L0=1e-3  Vl0=0
      settings: SourceProductBaseCode=PS
  Variable Inductor5.4 : spsVariableInductorLib/Variable Inductor  Commented=on  methode=Trapezoidal  Labsmin=0.1e-3  Initialize=off  iL0=0  L0=1e-3  Vl0=0
      settings: SourceProductBaseCode=PS
  Variable Inductor5.5 : spsVariableInductorLib/Variable Inductor  Commented=on  methode=Trapezoidal  Labsmin=0.1e-3  Initialize=off  iL0=0  L0=1e-3  Vl0=0
      settings: SourceProductBaseCode=PS
  Variable Inductor5.6 : spsVariableInductorLib/Variable Inductor  Commented=on  methode=Trapezoidal  Labsmin=0.1e-3  Initialize=off  iL0=0  L0=1e-3  Vl0=0
      settings: SourceProductBaseCode=PS
  abc to Alpha-Beta-Zero : spsabctoAlphaBetaZeroLib/abc to Alpha-Beta-Zero
      settings: SourceProductBaseCode=PS
  abc to dq0 : spsabctodq0Lib/abc to dq0  Alignment=90 degrees behind phase A axis
  powergui : spspowerguiLib/powergui  Priority=1  SimulationMode=Continuous  SampleTime=50e-6  frequency=60  Iterations=50  frequencyindice=60  Pbase=100e6  ErrMax=1e-4  UnitsV=kV  UnitsW=MW  buscounter=0  FunctionMessages=off  echomessages=off  EnableUseOfTLC=off  CurrentSourceSwitches=off  DisableSnubberDevices=off  DisableRonSwitches=off  DisableVfSwitches=off  DisplayEquations=off  AutomaticDiscreteSolvers=off  SolverType=Tustin/Backward Euler (TBE)  Interpol=off  ExternalGateDelay=off  methode=off  Ts=100  x0status=blocks  SPID=on  SwTol=0  HookPort=off  NonlinearTolerance=1e-4  nMaxIteration=100  ContinueOnMaxIteration=off  RestoreLinks=warning  ResistiveCurrentMeasurement=off  Frange=[0:2:500]  Ylog=off  Xlog=on  ShowGrid=off  save=off  variable=ZData  structure=0  ZoomFFT=off  StartTime=0.0  cycles=1  DisplayStyle=1  fundamental=60  FreqAxis=off  MaxFrequency=1000  frequencyindicesteady=1  RmsSteady=1  display=off
  VDC- : PMIOPort  Side=Left
  VDC-1 : PMIOPort  Port=2  Side=Left
  Connection Port : PMIOPort  Tag=PMCPort  Port=3  Side=Left
  Connection Port1 : PMIOPort  Tag=PMCPort  Port=4  Side=Left
  Connection Port2 : PMIOPort  Tag=PMCPort  Port=5  Side=Left
  Connection Port3 : PMIOPort  Tag=PMCPort  Port=6  Side=Right
  Connection Port4 : PMIOPort  Tag=PMCPort  Port=7  Side=Right
  Connection Port5 : PMIOPort  Tag=PMCPort  Port=8  Side=Right
  wires:
  Three-Phase V-I Measurement3/1 -> Scope/1
  [pwm1] -> IGBT/Diode/1
  Sum/1 -> PID Controller/1
  Alpha-Beta-Zero to dq0/1 -> Demux/1
  Demux/3 -> [Vq]
  Demux1/3 -> [Iq]
  [Vabc] -> abc to Alpha-Beta-Zero/1
  [alphabeta] -> Alpha-Beta-Zero to dq1/1
  Demux1/2 -> [Id]
  Integrator/1 -> [wt], Alpha-Beta-Zero to dq1/2
  Constant/1 -> Sum/2
  [Iabc] -> abc to dq0/1
  abc to dq0/1 -> Demux1/1
  [wt] -> abc to dq0/2
  [wt] -> Alpha-Beta-Zero to dq0/2
  Demux2/2 -> Sum/1
  PID Controller/1 -> Integrator/1
  abc to Alpha-Beta-Zero/1 -> Alpha-Beta-Zero to dq0/1, [alphabeta]
  Demux/2 -> [Vd]
  Alpha-Beta-Zero to dq1/1 -> Demux2/1
  [pwm2] -> IGBT/Diode8/1
  [pwm1] -> IGBT/Diode26/1
  Three-Phase V-I Measurement4/1 -> Scope1/1
  [pwm2] -> IGBT/Diode1/1
  [pwm3] -> IGBT/Diode2/1
  [pwm4] -> IGBT/Diode9/1
  [pwm4] -> IGBT/Diode3/1
  [pwm5] -> IGBT/Diode4/1
  [pwm3] -> IGBT/Diode11/1
  [pwm5] -> IGBT/Diode12/1
  [pwm6] -> IGBT/Diode5/1
  [A] -> IGBT/Diode7/1
  [A] -> IGBT/Diode13/1
  [pwm1] -> IGBT/Diode14/1
  [pwm2] -> IGBT/Diode23/1
  [pwm1] -> IGBT/Diode25/1
  [pwm2] -> IGBT/Diode15/1
  [pwm3] -> IGBT/Diode19/1
  [pwm4] -> IGBT/Diode24/1
  [pwm4] -> IGBT/Diode20/1
  [pwm3] -> IGBT/Diode17/1
  [pwm5] -> IGBT/Diode21/1
  [pwm6] -> IGBT/Diode16/1
  [pwm5] -> IGBT/Diode18/1
  [pwm6] -> IGBT/Diode22/1
  [pwm6] -> IGBT/Diode10/1
  [pwm6] -> Scope2/4
  [pwm4] -> Scope2/2
  Repeating Sequence/1 -> Relational Operator/2, Relational Operator1/2, Relational Operator2/2, Mux/4
  Sine Wave2/1 -> Mux/3, Relational Operator2/1
  Relational Operator/1 -> Logical Operator/1, [pwm1]
  Logical Operator2/1 -> [pwm2]
  Mux/1 -> Scope3/1
  Logical Operator1/1 -> [pwm6]
  Sine Wave/1 -> Relational Operator/1, Mux/1
  Relational Operator2/1 -> [pwm5], Logical Operator2/1
  Sine Wave1/1 -> Relational Operator1/1, Mux/2
  [pwm5] -> Scope2/5
  [pwm2] -> Scope2/6
  [pwm3] -> Scope2/3
  [pwm1] -> Scope2/1
  Logical Operator/1 -> [pwm4]
  Relational Operator1/1 -> [pwm3], Logical Operator1/1
  Constant2/1 -> Variable Inductor L4.3/1, Variable Inductor L4.2/1, Variable Inductor L4.1/1
  Constant3/1 -> Variable Inductor L6/1
  Constant4/1 -> Variable Inductor L6.1/1
  Constant5/1 -> Variable Inductor5.3/1, Variable Inductor5.2/1, Variable Inductor5.1/1
  Constant1/1 -> Variable Inductor5.6/1, Variable Inductor5.5/1, Variable Inductor5.4/1
  connections:
  IGBT/Diode/LConn1 -- Variable Inductor L6/LConn1 -- Series RLC Branch3/LConn1 -- IGBT/Diode4/LConn1 -- IGBT/Diode2/LConn1 -- VDC-/RConn1
  Series RLC Branch1/LConn1 -- Three-Phase Transformer (Two Windings)/RConn2 -- Variable Inductor L4.2/LConn1
  Series RLC Branch1/RConn1 -- Series RLC Branch/RConn1 -- Series RLC Branch2/RConn1 -- Ground1/LConn1 -- Diode8/LConn1 -- Diode13/RConn1 -- Diode11/RConn1 -- Diode10/LConn1 -- Diode12/RConn1 -- Diode9/LConn1 -- Series RLC Branch5/RConn1 -- Series RLC Branch6/LConn1 -- Three-Phase Transformer (Two Windings)1/LConn2 -- Three-Phase V-I Measurement4/RConn2 -- Three-Phase V-I Measurement4/RConn1 -- Three-Phase Transformer (Two Windings)1/LConn1 -- Three-Phase V-I Measurement4/RConn3 -- Three-Phase Transformer (Two Windings)1/LConn3 -- Ground/LConn1 -- Diode5/RConn1 -- Diode1/LConn1 -- Diode3/RConn1 -- Diode2/LConn1 -- Diode4/RConn1 -- Diode/LConn1 -- Series RLC Branch4/LConn1 -- Series RLC Branch3/RConn1
  Three-Phase Transformer (Two Windings)/RConn3 -- Series RLC Branch2/LConn1 -- Variable Inductor L4.3/LConn1
  IGBT/Diode25/RConn1 -- Diode11/LConn1 -- IGBT/Diode15/LConn1
  IGBT/Diode19/LConn1 -- IGBT/Diode21/LConn1 -- Variable Inductor L6/RConn1 -- IGBT/Diode7/LConn1 -- Series RLC Branch5/LConn1 -- IGBT/Diode14/LConn1
  Three-Phase Transformer (Two Windings)/RConn1 -- Series RLC Branch/LConn1 -- Variable Inductor L4.1/LConn1
  IGBT/Diode1/LConn1 -- IGBT/Diode26/RConn1 -- Diode3/LConn1
  Three-Phase V-I Measurement3/LConn1 -- IGBT/Diode18/LConn1 -- IGBT/Diode16/RConn1
  IGBT/Diode22/LConn1 -- Diode13/LConn1 -- IGBT/Diode18/RConn1
  Variable Inductor L6.1/LConn1 -- Series RLC Branch4/RConn1 -- IGBT/Diode5/RConn1 -- IGBT/Diode3/RConn1 -- IGBT/Diode1/RConn1 -- VDC-1/RConn1
  Series RLC Branch8/RConn1 -- IGBT/Diode13/LConn1 -- Diode7/LConn1
  IGBT/Diode5/LConn1 -- IGBT/Diode12/RConn1 -- Diode5/LConn1
  Variable Inductor5.6/RConn1 -- Three-Phase Transformer (Two Windings)/LConn3
  IGBT/Diode15/RConn1 -- IGBT/Diode22/RConn1 -- IGBT/Diode20/RConn1 -- Series RLC Branch6/RConn1 -- IGBT/Diode13/RConn1 -- Variable Inductor L6.1/RConn1
  Three-Phase V-I Measurement3/LConn2 -- IGBT/Diode17/LConn1 -- IGBT/Diode24/RConn1
  Three-Phase V-I Measurement4/LConn1 -- Variable Inductor5.1/RConn1
  Variable Inductor5.3/RConn1 -- Three-Phase V-I Measurement4/LConn3
  Series RLC Branch7/RConn1 -- Series RLC Branch8/LConn1
  Three-Phase V-I Measurement3/RConn2 -- Variable Inductor5.2/LConn1
  Diode9/RConn1 -- IGBT/Diode19/RConn1 -- IGBT/Diode24/LConn1
  Three-Phase V-I Measurement4/LConn2 -- Variable Inductor5.2/RConn1
  Three-Phase Transformer (Two Windings)1/RConn3 -- Connection Port5/RConn1
  IGBT/Diode8/RConn1 -- IGBT/Diode26/LConn1 -- Variable Inductor L4.1/RConn1
  IGBT/Diode23/RConn1 -- IGBT/Diode25/LConn1 -- Three-Phase V-I Measurement3/LConn3
  IGBT/Diode16/LConn1 -- Diode8/RConn1 -- IGBT/Diode21/RConn1
  Diode10/RConn1 -- IGBT/Diode14/RConn1 -- IGBT/Diode23/LConn1
  IGBT/Diode12/LConn1 -- IGBT/Diode10/RConn1 -- Variable Inductor L4.3/RConn1
  Three-Phase V-I Measurement3/RConn1 -- Variable Inductor5.1/LConn1
  Series RLC Branch7/LConn1 -- IGBT/Diode7/RConn1 -- Diode6/RConn1
  Diode2/RConn1 -- IGBT/Diode8/LConn1 -- IGBT/Diode/RConn1
  IGBT/Diode9/LConn1 -- IGBT/Diode2/RConn1 -- Diode1/RConn1
  IGBT/Diode17/RConn1 -- Diode12/LConn1 -- IGBT/Diode20/LConn1
  Variable Inductor L4.2/RConn1 -- IGBT/Diode9/RConn1 -- IGBT/Diode11/LConn1
  IGBT/Diode10/LConn1 -- IGBT/Diode4/RConn1 -- Diode/RConn1
  IGBT/Diode3/LConn1 -- IGBT/Diode11/RConn1 -- Diode4/LConn1
  Diode7/RConn1 -- Diode6/LConn1
  Variable Inductor5.3/LConn1 -- Three-Phase V-I Measurement3/RConn3
  Three-Phase Transformer (Two Windings)1/RConn2 -- Connection Port4/RConn1
  Three-Phase Transformer (Two Windings)1/RConn1 -- Connection Port3/RConn1
  Variable Inductor5.4/LConn1 -- Series RLC Branch9/LConn1 -- Connection Port/RConn1
  Variable Inductor5.6/LConn1 -- Series RLC Branch11/LConn1 -- Connection Port2/RConn1
  Variable Inductor5.5/LConn1 -- Series RLC Branch10/LConn1 -- Connection Port1/RConn1
  Variable Inductor5.5/RConn1 -- Three-Phase Transformer (Two Windings)/LConn2
  Variable Inductor5.4/RConn1 -- Three-Phase Transformer (Two Windings)/LConn1
  Series RLC Branch9/RConn1 -- Ground2/LConn1 -- Series RLC Branch10/RConn1 -- Series RLC Branch11/RConn1
